simulink model "htx_qp_torq_allocator"  (R2024b)
settings: Solver=FixedStepAuto  StartTime=0.0  StopTime=10.0  RelTol=1e-3
undefined symbols (not defined in the file): dspblkCoreblockFVToolHelper, gcbh, GR, R_wheel, rpm2rad_s
settings Model: Creator=lukec  LastModifiedBy=lukec
settings OptimizationCC: DefaultParameterBehavior=Inlined  EnhancedBackFolding=on  PassReuseOutputArgsAs=Individual arguments  ZeroExternalMemoryAtStartup=off  ZeroInternalMemoryAtStartup=off  OptimizeBlockOrder=speed  DifferentSizesBufferReuse=on  OptimizationCustomize=off  EfficientTunableParamExpr=on
settings DebuggingCC: ParameterTunabilityLossMsg=error
settings HardwareCC: ProdBitPerPointer=32  ProdBitPerSizeT=32  ProdBitPerPtrDiffT=32  ProdLargestAtomicInteger=Long  ProdLargestAtomicFloat=Double  ProdWordSize=32  ProdHWDeviceType=ARM Compatible->ARM Cortex-M
settings SFSimCC: MATLABDynamicMemAlloc=off
settings RTWCC: Description=Embedded Coder  SystemTargetFile=ert.tlc  GenCodeOnly=on  PackageGeneratedCodeAndArtifacts=on  TemplateMakefile=ert_default_tmf  Toolchain=CMake  TargetLang=C++
settings CodeAppCC: ForceParamTrailComments=on  IgnoreCustomStorageClasses=off  MaxIdLength=255  OperatorAnnotations=on  SimulinkDataObjDesc=on  SFDataObjDesc=on  InsertBlockDesc=on
settings ERTTargetCC: TargetLangStandard=C++17 (ISO)  CodeInterfacePackaging=C++ class  RootIOFormat=Structure reference  ERTCustomFileTemplate=example_file_process.tlc  ArrayContainerType=std::array

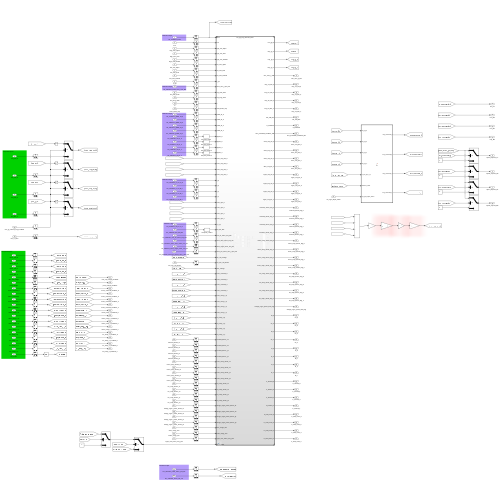
[thumbnail: Simulink's stored preview of the top-level diagram]
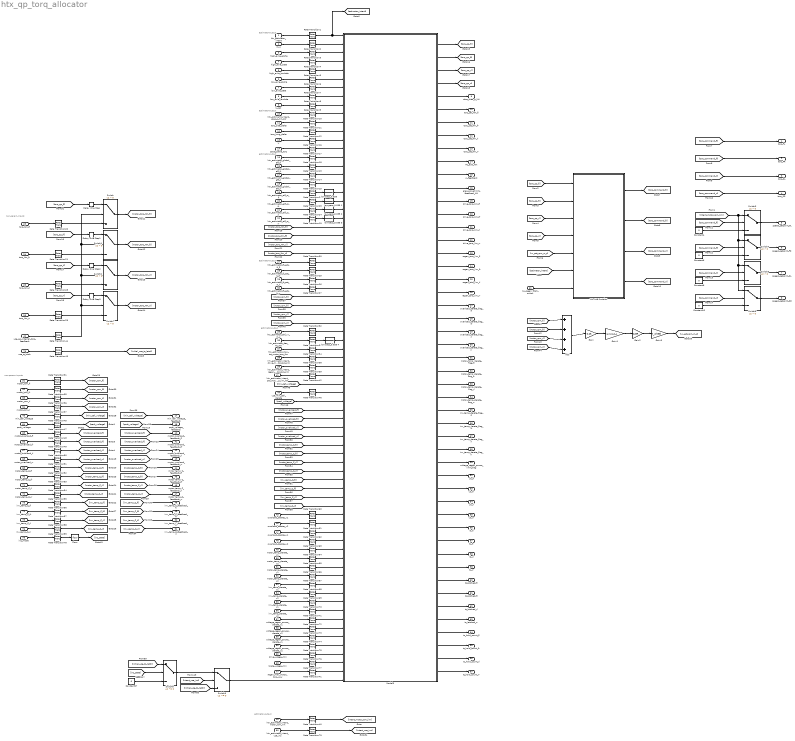
== system htx_qp_torq_allocator ==
  note: non-param-inputs
  note: estimator-output
  note: estimator-output
  note: estimator-output
  note: estimator-output
  note: estimator-output
  note: non-param-inputs
  note: estimator-output
  htx_estimator_intent : Inport
  mux : Inport  Port=2
  high_axle_alpha : Inport  Port=3
  high_axle_beta : Inport  Port=4
  high_axle_lambda : Inport  Port=5
  low_axle_alpha : Inport  Port=6
  low_axle_beta : Inport  Port=7
  low_axle_lambda : Inport  Port=8
  k_opt : Inport  Port=9
  htx_estimator_intent_elec_p_lim_kW : Inport  Port=10
  torq_side_delta : Inport  Port=11
  torq_long_delta : Inport  Port=12
  w : Inport  Port=13
  coast_brake_torq : Inport  Port=14
  htx_estimator_global_eff_fl : Inport  Port=15
  htx_estimator_global_eff_fr : Inport  Port=16
  htx_estimator_global_eff_rl : Inport  Port=17
  htx_estimator_global_eff_rr : Inport  Port=18
  htx_estimator_ekf_sr_fl : Inport  Port=19
  htx_estimator_ekf_sr_fr : Inport  Port=20
  htx_estimator_ekf_sr_rl : Inport  Port=21
  htx_estimator_ekf_sr_rr : Inport  Port=22
  torq_Nm_fl : Inport  Port=23
  torq_Nm_fr : Inport  Port=24
  torq_Nm_rl : Inport  Port=25
  torq_Nm_rr : Inport  Port=26
  htx_estimator_fz_est_N_fl : Inport  Port=27
  htx_estimator_fz_est_N_fr : Inport  Port=28
  htx_estimator_fz_est_N_rl : Inport  Port=29
  htx_estimator_fz_est_N_rr : Inport  Port=30
  motor_rpm_fl : Inport  Port=31
  motor_rpm_fr : Inport  Port=32
  motor_rpm_rl : Inport  Port=33
  motor_rpm_rr : Inport  Port=34
  htx_estimator_ekf_vx_m_s : Inport  Port=35
  htx_estimator_des_Mz_Nm : Inport  Port=36
  htx_estimator_max_tot_motor_torq_Nm : Inport  Port=37
  htx_estimator_intent_drive_motor_torq_lim : Inport  Port=38
  htx_estimator_intent_regen_motor_torq_lim : Inport  Port=39
  htx_estimator_intent_motor_rpm_lim : Inport  Port=40
  htx_estimator_intent_per_motor_elec_p_lim_kW : Inport  Port=41
  use_qp_internal_torq_feedback : Inport  Port=42
  min_cell_voltage : Inport  Port=43
  use_min_cell_derate : Inport  Port=44
  overload_derate_x1 : Inport  Port=45
  overload_derate_x2 : Inport  Port=46
  overload_derate_y1 : Inport  Port=47
  overload_derate_y2 : Inport  Port=48
  motor_temp_derate_x1 : Inport  Port=49
  motor_temp_derate_x2 : Inport  Port=50
  motor_temp_derate_y1 : Inport  Port=51
  motor_temp_derate_y2 : Inport  Port=52
  inv_temp_derate_x1 : Inport  Port=53
  inv_temp_derate_x2 : Inport  Port=54
  inv_temp_derate_y1 : Inport  Port=55
  inv_temp_derate_y2 : Inport  Port=56
  voltage_regen_power_derate_x1 : Inport  Port=57
  voltage_regen_power_derate_x2 : Inport  Port=58
  voltage_regen_power_derate_y1 : Inport  Port=59
  voltage_regen_power_derate_y2 : Inport  Port=60
  no_regen_5kph_switch : Inport  Port=61
  drive_usage_min : Inport  Port=62
  brake_usage_min : Inport  Port=63
  pack_voltage : Inport  Port=64
  motor_overload_fl : Inport  Port=65
  motor_overload_fr : Inport  Port=66
  motor_overload_rl : Inport  Port=67
  motor_overload_rr : Inport  Port=68
  motor_temp_C_fl : Inport  Port=69
  motor_temp_C_fr : Inport  Port=70
  motor_temp_C_rl : Inport  Port=71
  motor_temp_C_rr : Inport  Port=72
  inv_temp_C_fl : Inport  Port=73
  inv_temp_C_fr : Inport  Port=74
  inv_temp_C_rl : Inport  Port=75
  inv_temp_C_rr : Inport  Port=76
  regen_max_motor_torq_yaw : Inport  Port=77
  use_tc_latch : Inport  Port=78
  ins_mode : Inport  Port=79
  htx_estimator_intent_use_ins : Inport  Port=80
  Add : Sum  Inputs=++++
  Constant{4,6,8,10,27} (5 alike) : Constant  Value=0
  Delay One Step{,1..3} (4 alike) : Delay  DelayLength=1  SampleTime=0.004
  Floor : Rounding
  Gain : Gain  Gain=0.25
  Gain1 : Gain  Gain=rpm2rad_s
  Gain2 : Gain  Gain=1/GR
  Gain3 : Gain  Gain=R_wheel
  MATLAB Function : MATLAB Function  TreatAsAtomicUnit=on
  Model5 : ModelReference  ModelNameDialog=htx_qp_torq_allocator_base.slx  SimulationMode=Normal  ModelReferenceVersion=1.61
  Rate Transition{1..79} (79 alike) : RateTransition  OutPortSampleTime=0.004
  Switch{,1..7} (8 alike) : Switch  Criteria=u2 > Threshold  SaturateOnIntegerOverflow=off  InputSameDT=off
  Switch8 : Switch  Criteria=u2 ~= 0  SaturateOnIntegerOverflow=off  InputSameDT=off
  Switch9 : Switch  Criteria=u2 ~= 0  SaturateOnIntegerOverflow=off  InputSameDT=off
  low-pass_0.035 {,1..4} (5 alike) : DiscreteTransferFcn  LoadFcn=dspblkCoreblockFVToolHelper(gcbh,'load');  Numerator=[0, 0.1143]  Denominator=[1, -0.8857]
      settings: CopyFcn=dspblkCoreblockFVToolHelper(gcbh,'copy');  DeleteFcn=dspblkCoreblockFVToolHelper(gcbh,'close');  ModelCloseFcn=dspblkCoreblockFVToolHelper(gcbh,'close');  PreSaveFcn=dspblkCoreblockFVToolHelper(gcbh,'presave');  PostSaveFcn=dspblkCoreblockFVToolHelper(gcbh,'postsave');  CloseFcn=dspblkCoreblockFVToolHelper(gcbh,'close');
  torq_FL : Outport
  torq_FR : Outport  Port=2
  torq_RL : Outport  Port=3
  torq_RR : Outport  Port=4
  speed_setpoint_FL : Outport  Port=5
  speed_setpoint_FR : Outport  Port=6
  speed_setpoint_RL : Outport  Port=7
  speed_setpoint_RR : Outport  Port=8
  elec_theo_p_kW : Outport  Port=9
  torq_sat_Nm_fl : Outport  Port=10
  torq_sat_Nm_fr : Outport  Port=11
  torq_sat_Nm_rl : Outport  Port=12
  torq_sat_Nm_rr : Outport  Port=13
  Mz_add_Nm : Outport  Port=14
  w_feedback : Outport  Port=15
  elec_powerlimit_feedback_kW : Outport  Port=16
  min_cell_voltage_feedback : Outport  Port=17
  pack_voltage_feedback : Outport  Port=18
  drive_torq_lim_fl : Outport  Port=19
  drive_torq_lim_fr : Outport  Port=20
  drive_torq_lim_rl : Outport  Port=21
  drive_torq_lim_rr : Outport  Port=22
  regen_torq_lim_fl : Outport  Port=23
  regen_torq_lim_fr : Outport  Port=24
  regen_torq_lim_rl : Outport  Port=25
  regen_torq_lim_rr : Outport  Port=26
  overload_derate_flag_fl : Outport  Port=27
  overload_derate_flag_fr : Outport  Port=28
  overload_derate_flag_rl : Outport  Port=29
  overload_derate_flag_rr : Outport  Port=30
  motor_temp_derate_flag_fl : Outport  Port=31
  motor_temp_derate_flag_fr : Outport  Port=32
  motor_temp_derate_flag_rl : Outport  Port=33
  motor_temp_derate_flag_rr : Outport  Port=34
  inv_temp_derate_flag_fl : Outport  Port=35
  inv_temp_derate_flag_fr : Outport  Port=36
  inv_temp_derate_flag_rl : Outport  Port=37
  inv_temp_derate_flag_rr : Outport  Port=38
  voltage_regen_power_limit_flag : Outport  Port=39
  motor_overload_feedback_fl : Outport  Port=40
  motor_overload_feedback_fr : Outport  Port=41
  motor_overload_feedback_rl : Outport  Port=42
  motor_overload_feedback_rr : Outport  Port=43
  motor_temp_C_feedback_fl : Outport  Port=44
  motor_temp_C_feedback_fr : Outport  Port=45
  motor_temp_C_feedback_rl : Outport  Port=46
  motor_temp_C_feedback_rr : Outport  Port=47
  inv_temp_C_feedback_fl : Outport  Port=48
  inv_temp_C_feedback_fr : Outport  Port=49
  inv_temp_C_feedback_rl : Outport  Port=50
  inv_temp_C_feedback_rr : Outport  Port=51
  ub_fl : Outport  Port=52
  ub_fr : Outport  Port=53
  ub_rl : Outport  Port=54
  ub_rr : Outport  Port=55
  lb_fl : Outport  Port=56
  lb_fr : Outport  Port=57
  lb_rl : Outport  Port=58
  lb_rr : Outport  Port=59
  tc_latched_fl : Outport  Port=60
  tc_latched_fr : Outport  Port=61
  tc_latched_rl : Outport  Port=62
  tc_latched_rr : Outport  Port=63
  tc_hold_count_fl : Outport  Port=64
  tc_hold_count_fr : Outport  Port=65
  tc_hold_count_rl : Outport  Port=66
  tc_hold_count_rr : Outport  Port=67
  wires:
  htx_estimator_intent/1 -> Rate Transition1/1
  mux/1 -> Rate Transition2/1
  high_axle_alpha/1 -> Rate Transition3/1
  high_axle_beta/1 -> Rate Transition4/1
  high_axle_lambda/1 -> Rate Transition5/1
  low_axle_alpha/1 -> Rate Transition6/1
  low_axle_beta/1 -> Rate Transition7/1
  low_axle_lambda/1 -> Rate Transition8/1
  k_opt/1 -> Rate Transition9/1
  htx_estimator_intent_elec_p_lim_kW/1 -> Rate Transition10/1
  torq_side_delta/1 -> Rate Transition11/1
  torq_long_delta/1 -> Rate Transition12/1
  w/1 -> Rate Transition16/1
  coast_brake_torq/1 -> Rate Transition17/1
  htx_estimator_global_eff_fl/1 -> Rate Transition18/1
  htx_estimator_global_eff_fr/1 -> Rate Transition13/1
  htx_estimator_global_eff_rl/1 -> Rate Transition14/1
  htx_estimator_global_eff_rr/1 -> Rate Transition15/1
  htx_estimator_ekf_sr_fl/1 -> Rate Transition22/1
  htx_estimator_ekf_sr_fr/1 -> Rate Transition23/1
  htx_estimator_ekf_sr_rl/1 -> Rate Transition24/1
  htx_estimator_ekf_sr_rr/1 -> Rate Transition19/1
  torq_Nm_fl/1 -> Rate Transition20/1
  torq_Nm_fr/1 -> Rate Transition21/1
  torq_Nm_rl/1 -> Rate Transition28/1
  torq_Nm_rr/1 -> Rate Transition29/1
  htx_estimator_fz_est_N_fl/1 -> Rate Transition30/1
  htx_estimator_fz_est_N_fr/1 -> Rate Transition25/1
  htx_estimator_fz_est_N_rl/1 -> Rate Transition26/1
  htx_estimator_fz_est_N_rr/1 -> Rate Transition27/1
  motor_rpm_fl/1 -> Rate Transition31/1
  motor_rpm_fr/1 -> Rate Transition35/1
  motor_rpm_rl/1 -> Rate Transition36/1
  motor_rpm_rr/1 -> Rate Transition37/1
  htx_estimator_ekf_vx_m_s/1 -> Rate Transition32/1
  htx_estimator_des_Mz_Nm/1 -> Rate Transition33/1
  htx_estimator_max_tot_motor_torq_Nm/1 -> Rate Transition34/1
  htx_estimator_intent_drive_motor_torq_lim/1 -> Rate Transition38/1
  htx_estimator_intent_regen_motor_torq_lim/1 -> Rate Transition39/1
  Rate Transition1/1 -> [estimator_intent], Model5/1
  Rate Transition2/1 -> Model5/2
  Rate Transition3/1 -> Model5/3
  Rate Transition6/1 -> Model5/6
  Rate Transition5/1 -> Model5/5
  Rate Transition4/1 -> Model5/4
  Rate Transition8/1 -> Model5/8
  Rate Transition10/1 -> Model5/10
  Rate Transition11/1 -> Model5/11
  Rate Transition9/1 -> Model5/9
  Rate Transition12/1 -> Model5/12
  Rate Transition7/1 -> Model5/7
  Rate Transition14/1 -> Model5/17
  Rate Transition15/1 -> Model5/18
  Rate Transition16/1 -> Model5/13
  Rate Transition17/1 -> Model5/14
  Rate Transition13/1 -> Model5/16
  Rate Transition18/1 -> Model5/15
  Rate Transition19/1 -> low-pass_0.035 3/1
  Rate Transition24/1 -> low-pass_0.035 2/1
  Rate Transition22/1 -> "low-pass_0.035 "/1
  Rate Transition23/1 -> low-pass_0.035 1/1
  Rate Transition26/1 -> Model5/29
  Rate Transition27/1 -> Model5/30
  Rate Transition30/1 -> Model5/27
  Rate Transition25/1 -> Model5/28
  Rate Transition32/1 -> Model5/35
  Rate Transition33/1 -> low-pass_0.035 4/1
  Rate Transition34/1 -> Model5/37
  Rate Transition39/1 -> Model5/39
  Rate Transition38/1 -> Model5/38
  htx_estimator_intent_motor_rpm_lim/1 -> Rate Transition40/1
  Rate Transition40/1 -> [intent_motor_rpm_lim]
  Constant8/1 -> Switch5/3
  Switch4/1 -> speed_setpoint_FR/1
  Switch3/1 -> speed_setpoint_FL/1
  [torq_command_fr] -> Switch4/2
  [intent_motor_rpm_lim] -> Switch6/1, Switch5/1, Switch4/1, Switch3/1
  Switch6/1 -> speed_setpoint_RR/1
  [torq_command_rr] -> Switch6/2
  Constant4/1 -> Switch3/3
  [torq_command_rl] -> Switch5/2
  Constant6/1 -> Switch4/3
  Constant10/1 -> Switch6/3
  [torq_command_fl] -> Switch3/2
  Switch5/1 -> speed_setpoint_RL/1
  Model5/5 -> elec_theo_p_kW/1
  Model5/6 -> torq_sat_Nm_fl/1
  Model5/7 -> torq_sat_Nm_fr/1
  Model5/8 -> torq_sat_Nm_rl/1
  Model5/9 -> torq_sat_Nm_rr/1
  Model5/10 -> Mz_add_Nm/1
  [estimator_intent] -> MATLAB Function/6(estimator_intent)
  MATLAB Function/1(torq_command_fl) -> [torq_command_fl]
  MATLAB Function/2(torq_command_fr) -> [torq_command_fr]
  MATLAB Function/3(torq_command_rl) -> [torq_command_rl]
  MATLAB Function/4(torq_command_rr) -> [torq_command_rr]
  [torq_command_fl] -> torq_FL/1
  [torq_command_fr] -> torq_FR/1
  [torq_command_rl] -> torq_RL/1
  [torq_command_rr] -> torq_RR/1
  Model5/11 -> w_feedback/1
  htx_estimator_intent_per_motor_elec_p_lim_kW/1 -> Rate Transition42/1
  use_qp_internal_torq_feedback/1 -> Rate Transition44/1
  Rate Transition44/1 -> Switch2/2, Switch/2, Switch1/2, Switch7/2
  Rate Transition20/1 -> Switch/3
  [torq_qp_fl] -> Delay One Step/1
  Delay One Step/1 -> Switch/1
  Delay One Step1/1 -> Switch1/1
  Delay One Step2/1 -> Switch2/1
  Delay One Step3/1 -> Switch7/1
  [torq_qp_fr] -> Delay One Step1/1
  [torq_qp_rl] -> Delay One Step2/1
  [torq_qp_rr] -> Delay One Step3/1
  Rate Transition21/1 -> Switch1/3
  Rate Transition28/1 -> Switch2/3
  Rate Transition29/1 -> Switch7/3
  Model5/12 -> elec_powerlimit_feedback_kW/1
  min_cell_voltage/1 -> Rate Transition45/1
  use_min_cell_derate/1 -> Rate Transition46/1
  Switch/1 -> [motor_torq_Nm_fl]
  Switch1/1 -> [motor_torq_Nm_fr]
  Switch2/1 -> [motor_torq_Nm_rl]
  Switch7/1 -> [motor_torq_Nm_rr]
  [motor_torq_Nm_fl] -> Model5/23
  [motor_torq_Nm_fr] -> Model5/24
  [motor_torq_Nm_rr] -> Model5/26
  [motor_torq_Nm_rl] -> Model5/25
  overload_derate_x1/1 -> Rate Transition60/1
  overload_derate_x2/1 -> Rate Transition61/1
  overload_derate_y1/1 -> Rate Transition62/1
  overload_derate_y2/1 -> Rate Transition63/1
  motor_temp_derate_x1/1 -> Rate Transition64/1
  motor_temp_derate_x2/1 -> Rate Transition65/1
  motor_temp_derate_y1/1 -> Rate Transition66/1
  motor_temp_derate_y2/1 -> Rate Transition67/1
  inv_temp_derate_x1/1 -> Rate Transition68/1
  inv_temp_derate_x2/1 -> Rate Transition69/1
  inv_temp_derate_y1/1 -> Rate Transition70/1
  inv_temp_derate_y2/1 -> Rate Transition71/1
  voltage_regen_power_derate_x1/1 -> Rate Transition72/1
  voltage_regen_power_derate_x2/1 -> Rate Transition73/1
  voltage_regen_power_derate_y1/1 -> Rate Transition74/1
  voltage_regen_power_derate_y2/1 -> Rate Transition75/1
  no_regen_5kph_switch/1 -> MATLAB Function/7(no_regen_5kph_switch)
  Model5/1 -> [torq_qp_fl]
  Model5/2 -> [torq_qp_fr]
  Model5/3 -> [torq_qp_rl]
  Model5/4 -> [torq_qp_rr]
  drive_usage_min/1 -> Rate Transition76/1
  brake_usage_min/1 -> Rate Transition77/1
  [torq_qp_fl] -> MATLAB Function/1(torq_qp_fl)
  [torq_qp_fr] -> MATLAB Function/2(torq_qp_fr)
  [torq_qp_rl] -> MATLAB Function/3(torq_qp_rl)
  [torq_qp_rr] -> MATLAB Function/4(torq_qp_rr)
  motor_temp_C_rl/1 -> Rate Transition54/1
  inv_temp_C_fr/1 -> Rate Transition57/1
  pack_voltage/1 -> Rate Transition47/1
  motor_overload_fr/1 -> Rate Transition49/1
  motor_overload_rr/1 -> Rate Transition51/1
  motor_overload_rl/1 -> Rate Transition50/1
  motor_temp_C_fr/1 -> Rate Transition53/1
  motor_temp_C_rr/1 -> Rate Transition55/1
  inv_temp_C_fl/1 -> Rate Transition56/1
  motor_temp_C_fl/1 -> Rate Transition52/1
  inv_temp_C_rl/1 -> Rate Transition58/1
  motor_overload_fl/1 -> Rate Transition48/1
  inv_temp_C_rr/1 -> Rate Transition59/1
  Rate Transition47/1 -> [pack_voltage]
  Rate Transition48/1 -> [motor_overload_fl]
  Rate Transition59/1 -> [inv_temp_C_rr]
  Rate Transition58/1 -> [inv_temp_C_rl]
  Rate Transition57/1 -> [inv_temp_C_fr]
  Rate Transition56/1 -> [inv_temp_C_fl]
  Rate Transition55/1 -> [motor_temp_C_rr]
  Rate Transition54/1 -> [motor_temp_C_rl]
  Rate Transition53/1 -> [motor_temp_C_fr]
  Rate Transition52/1 -> [motor_temp_C_fl]
  Rate Transition51/1 -> [motor_overload_rr]
  Rate Transition50/1 -> [motor_overload_rl]
  Rate Transition49/1 -> [motor_overload_fr]
  [motor_overload_fl] -> motor_overload_feedback_fl/1
  [motor_overload_fr] -> motor_overload_feedback_fr/1
  [motor_overload_rl] -> motor_overload_feedback_rl/1
  [motor_overload_rr] -> motor_overload_feedback_rr/1
  [motor_temp_C_fl] -> motor_temp_C_feedback_fl/1
  [motor_temp_C_fr] -> motor_temp_C_feedback_fr/1
  [motor_temp_C_rl] -> motor_temp_C_feedback_rl/1
  [motor_temp_C_rr] -> motor_temp_C_feedback_rr/1
  [inv_temp_C_fl] -> inv_temp_C_feedback_fl/1
  [inv_temp_C_fr] -> inv_temp_C_feedback_fr/1
  [inv_temp_C_rl] -> inv_temp_C_feedback_rl/1
  [inv_temp_C_rr] -> inv_temp_C_feedback_rr/1
  [pack_voltage] -> pack_voltage_feedback/1
  [min_cell_voltage] -> min_cell_voltage_feedback/1
  Rate Transition31/1 -> [motor_rpm_fl]
  Rate Transition37/1 -> [motor_rpm_rr]
  Rate Transition36/1 -> [motor_rpm_rl]
  Rate Transition35/1 -> [motor_rpm_fr]
  [motor_rpm_fl] -> Model5/31
  [motor_rpm_fr] -> Model5/32
  [motor_rpm_rl] -> Model5/33
  [motor_rpm_rr] -> Model5/34
  [motor_rpm_fl] -> Add/1
  [motor_rpm_fr] -> Add/2
  [motor_rpm_rl] -> Add/3
  [motor_rpm_rr] -> Add/4
  Add/1 -> Gain/1
  Gain/1 -> Gain1/1
  Gain1/1 -> Gain2/1
  Gain2/1 -> Gain3/1
  Gain3/1 -> [vx_est_rpm_m_s]
  [vx_est_rpm_m_s] -> MATLAB Function/5(vx_est_rpm_m_s)
  Rate Transition42/1 -> Model5/40
  [min_cell_voltage] -> Model5/41
  Rate Transition46/1 -> Model5/42
  Rate Transition45/1 -> [min_cell_voltage]
  [pack_voltage] -> Model5/43
  [motor_overload_fl] -> Model5/44
  [motor_overload_fr] -> Model5/45
  [motor_overload_rl] -> Model5/46
  [motor_overload_rr] -> Model5/47
  [inv_temp_C_fl] -> Model5/52
  [motor_temp_C_fl] -> Model5/48
  [motor_temp_C_fr] -> Model5/49
  [motor_temp_C_rl] -> Model5/50
  [motor_temp_C_rr] -> Model5/51
  [inv_temp_C_fr] -> Model5/53
  [inv_temp_C_rl] -> Model5/54
  [inv_temp_C_rr] -> Model5/55
  Rate Transition60/1 -> Model5/56
  Rate Transition61/1 -> Model5/57
  Rate Transition62/1 -> Model5/58
  Rate Transition63/1 -> Model5/59
  Rate Transition64/1 -> Model5/60
  Rate Transition65/1 -> Model5/61
  Rate Transition66/1 -> Model5/62
  Rate Transition67/1 -> Model5/63
  Rate Transition68/1 -> Model5/64
  Rate Transition69/1 -> Model5/65
  Rate Transition70/1 -> Model5/66
  Rate Transition71/1 -> Model5/67
  Rate Transition72/1 -> Model5/68
  Rate Transition73/1 -> Model5/69
  Rate Transition74/1 -> Model5/70
  Rate Transition75/1 -> Model5/71
  Rate Transition76/1 -> Model5/72
  Rate Transition77/1 -> Model5/73
  regen_max_motor_torq_yaw/1 -> Rate Transition41/1
  Rate Transition41/1 -> Model5/74
  use_tc_latch/1 -> Rate Transition43/1
  Model5/13 -> drive_torq_lim_fl/1
  Model5/14 -> drive_torq_lim_fr/1
  Model5/15 -> drive_torq_lim_rl/1
  Model5/16 -> drive_torq_lim_rr/1
  Model5/17 -> regen_torq_lim_fl/1
  Model5/18 -> regen_torq_lim_fr/1
  Model5/19 -> regen_torq_lim_rl/1
  Model5/20 -> regen_torq_lim_rr/1
  Model5/21 -> overload_derate_flag_fl/1
  Model5/22 -> overload_derate_flag_fr/1
  Model5/23 -> overload_derate_flag_rl/1
  Model5/24 -> overload_derate_flag_rr/1
  Model5/25 -> motor_temp_derate_flag_fl/1
  Model5/26 -> motor_temp_derate_flag_fr/1
  Model5/27 -> motor_temp_derate_flag_rl/1
  Model5/28 -> motor_temp_derate_flag_rr/1
  Model5/29 -> inv_temp_derate_flag_fl/1
  Model5/30 -> inv_temp_derate_flag_fr/1
  Model5/31 -> inv_temp_derate_flag_rl/1
  Model5/32 -> inv_temp_derate_flag_rr/1
  Model5/33 -> voltage_regen_power_limit_flag/1
  Model5/34 -> ub_fl/1
  Model5/35 -> ub_fr/1
  Model5/36 -> ub_rl/1
  Model5/37 -> ub_rr/1
  Model5/38 -> lb_fl/1
  Model5/39 -> lb_fr/1
  Model5/40 -> lb_rl/1
  Model5/41 -> lb_rr/1
  Model5/42 -> tc_latched_fl/1
  Model5/45 -> tc_latched_rr/1
  Model5/46 -> tc_hold_count_fl/1
  Model5/47 -> tc_hold_count_fr/1
  Model5/48 -> tc_hold_count_rl/1
  Model5/49 -> tc_hold_count_rr/1
  Model5/44 -> tc_latched_rl/1
  Model5/43 -> tc_latched_fr/1
  ins_mode/1 -> Rate Transition78/1
  Rate Transition78/1 -> Floor/1
  Rate Transition43/1 -> [initial_use_tc_latch]
  Switch9/1 -> Model5/75
  [initial_use_tc_latch] -> Switch8/1
  Constant27/1 -> Switch8/3
  [ins_state] -> Switch8/2
  Switch8/1 -> Switch9/1
  [initial_use_tc_latch] -> Switch9/3
  [intent_use_ins] -> Switch9/2
  htx_estimator_intent_use_ins/1 -> Rate Transition79/1
  Rate Transition79/1 -> [intent_use_ins]
  Floor/1 -> [ins_state]
  "low-pass_0.035 "/1 -> Model5/19
  low-pass_0.035 1/1 -> Model5/20
  low-pass_0.035 2/1 -> Model5/21
  low-pass_0.035 3/1 -> Model5/22
  low-pass_0.035 4/1 -> Model5/36

== matlab function htx_qp_torq_allocator/MATLAB Function ==
  data: torq_qp_fl input; torq_command_fl output; torq_qp_fr input; torq_qp_rl input; torq_qp_rr input; vx_est_rpm_m_s input; torq_command_fr output; torq_command_rl output; torq_command_rr output; estimator_intent input; no_regen_5kph_switch input
function [torq_command_fl, torq_command_fr, torq_command_rl, torq_command_rr] = fcn(torq_qp_fl, torq_qp_fr, torq_qp_rl, torq_qp_rr, vx_est_rpm_m_s, estimator_intent, no_regen_5kph_switch)

    switch no_regen_5kph_switch
        case 1
        case 0
        otherwise
            no_regen_5kph_switch = 1;
    end

    if no_regen_5kph_switch == 0
        torq_command_fl = torq_qp_fl;
        torq_command_fr = torq_qp_fr;
        torq_command_rl = torq_qp_rl;
        torq_command_rr = torq_qp_rr;
    else

        regen_derate_speed = 10/3.6;
        no_regen_speed = 5/3.6;
    
        if vx_est_rpm_m_s < no_regen_speed
            
            % speed under 5 KPH
    
            if estimator_intent < 0
    
                % Attempting to brake, cut regen
                torq_command_fl = 0;
                torq_command_fr = 0;
                torq_command_rl = 0;
                torq_command_rr = 0;
    
            else
    
                % passthrough
                torq_command_fl = torq_qp_fl;
                torq_command_fr = torq_qp_fr;
                torq_command_rl = torq_qp_rl;
                torq_command_rr = torq_qp_rr;
    
            end
    
        elseif vx_est_rpm_m_s < regen_derate_speed && vx_est_rpm_m_s > no_regen_speed
    
            % speed greater than 5 KPH and less than 10 KPH
    
            if estimator_intent < 0
    
                % Attempting to brake
                gain = interp1([no_regen_speed, regen_derate_speed], [0, 1], vx_est_rpm_m_s);
    
                torq_command_fl = torq_qp_fl * gain;
                torq_command_fr = torq_qp_fr * gain;
                torq_command_rl = torq_qp_rl * gain;
                torq_command_rr = torq_qp_rr * gain;
    
            else
    
                % passthrough
                torq_command_fl = torq_qp_fl;
                torq_command_fr = torq_qp_fr;
                torq_command_rl = torq_qp_rl;
                torq_command_rr = torq_qp_rr;
    
            end
    
        else
            
            % speed above 10 KPH
            torq_command_fl = torq_qp_fl;
            torq_command_fr = torq_qp_fr;
            torq_command_rl = torq_qp_rl;
            torq_command_rr = torq_qp_rr;
    
        end

    end
